simulink model "Subsystem"  (R2020b)
settings: Solver=VariableStepAuto  StartTime=0.0  StopTime=10.0  RelTol=1e-3
settings Model: Creator=dell  LastModifiedBy=dell
settings DataIOCC: SaveOutput=off  SaveTime=off

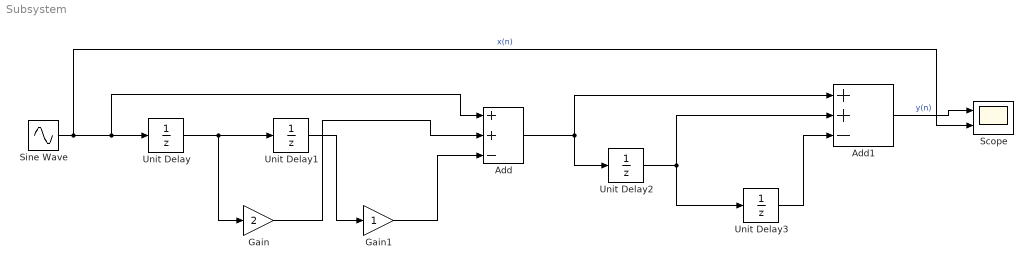
== system Subsystem ==
  Add : Sum  Inputs=++-
  Add1 : Sum  Inputs=++-
  Gain : Gain  Gain=2
  Gain1 : Gain
  Scope : Scope  NumInputPorts=2
  Sine Wave : Sin  SampleTime=0
  Unit Delay{,1..3} (4 alike) : UnitDelay  SampleTime=-1  HasFrameUpgradeWarning=on
  wires:
  Add/1 -> Unit Delay2/1, Add1/1
  Sine Wave/1 -> Scope/2, Unit Delay/1, Add/1  "x(n)"
  Gain/1 -> Add/2
  Add1/1 -> Scope/1  "y(n)"
  Gain1/1 -> Add/3
  Unit Delay2/1 -> Unit Delay3/1, Add1/2
  Unit Delay1/1 -> Gain1/1
  Unit Delay3/1 -> Add1/3
  Unit Delay/1 -> Unit Delay1/1, Gain/1
